simulink model "step_frequence_signal"  (R2024b)
settings: Solver=VariableStepAuto  StartTime=0.0  StopTime=0.4e-6  RelTol=1e-3
settings Model: Creator=brunoalexandrefraga  LastModifiedBy=brunoalexandrefraga

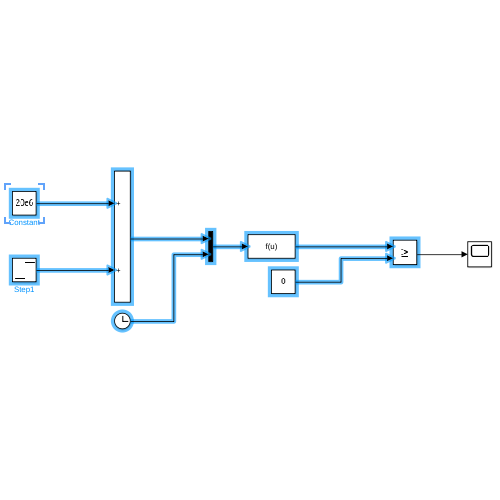
[thumbnail: Simulink's stored preview of the top-level diagram]
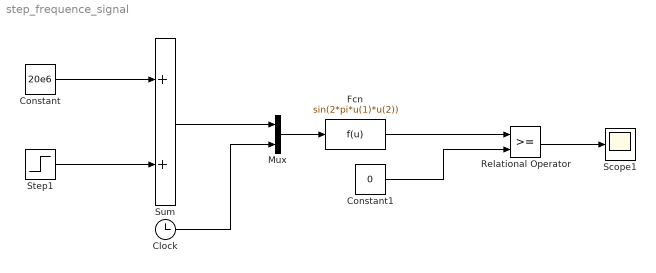
== system step_frequence_signal ==
  Clock : Clock
  Constant : Constant  Value=20e6  SampleTime=1e-9
  Constant1 : Constant  Value=0
  Fcn : Fcn  Expr=sin(2*pi*u(1)*u(2))
  Mux : Mux  Inputs=2
  Relational Operator : RelationalOperator  OutDataTypeStr=boolean  RndMeth=Simplest  InputSameDT=off
  Scope1 : Scope
  Step1 : Step  Time=0.2e-6  After=20e6  SampleTime=1e-9
  Sum : Sum
  wires:
  Sum/1 -> Mux/1
  Step1/1 -> Sum/2
  Constant/1 -> Sum/1
  Clock/1 -> Mux/2
  Mux/1 -> Fcn/1
  Constant1/1 -> Relational Operator/2
  Fcn/1 -> Relational Operator/1
  Relational Operator/1 -> Scope1/1
